simulink model "PID_controller"  (R2020a)
settings: Solver=VariableStepAuto  StartTime=0.0  StopTime=10.0  RelTol=1e-3
values from neighbouring files (symbols this model uses):
  kd = 1    [workspace_data.mat]
  ki = 40    [workspace_data.mat]
  kp = 800    [workspace_data.mat]
settings Model: Creator=shweta  LastModifiedBy=shweta
settings DataIOCC: SaveOutput=off  SaveTime=off

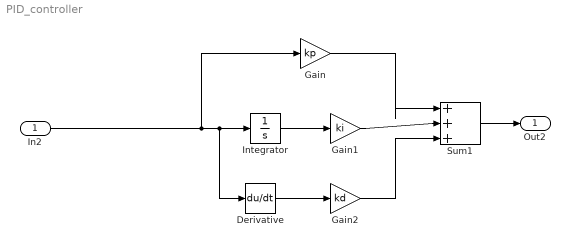
== system PID_controller ==
  In2 : Inport  OutDataTypeStr=double  PortDimensions=1  SampleTime=0
  Derivative : Derivative
  Gain : Gain  Gain=kp
  Gain1 : Gain  Gain=ki
  Gain2 : Gain  Gain=kd
  Integrator : Integrator
  Sum1 : Sum  Inputs=|+++
  Out2 : Outport  OutDataTypeStr=double  PortDimensions=1  SampleTime=0
  wires:
  Gain2/1 -> Sum1/3
  Sum1/1 -> Out2/1
  Integrator/1 -> Gain1/1
  Gain1/1 -> Sum1/2
  In2/1 -> Integrator/1, Derivative/1, Gain/1
  Derivative/1 -> Gain2/1
  Gain/1 -> Sum1/1
